simulink model "ADRC_2RD"  (Simulink 7.6)
settings: Solver=ode45  StartTime=0.0  StopTime=20  RelTol=1e-3
libraries: ADRC x3
settings Model: Creator=Administrator  LastModifiedBy=Administrator
settings DebuggingCC: AlgebraicLoopMsg=none  SolverPrmCheckMsg=none

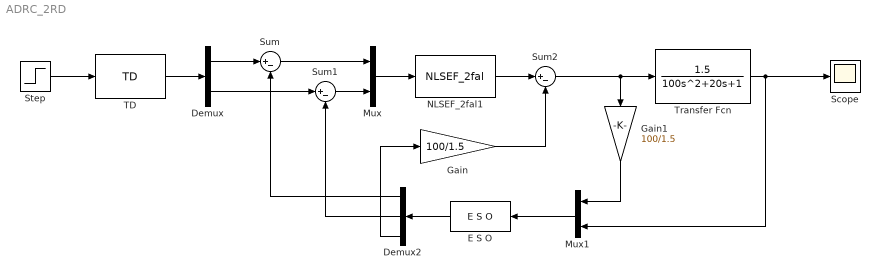
== system ADRC_2RD ==
  Demux : Demux  Outputs=2
  Demux2 : Demux  Outputs=3
  E S O : ADRC/ESO/E S O  Delta=0.1  h2=0.1  BB=[100,34,32]
  Gain : Gain  Gain=100/1.5
  Gain1 : Gain  Gain=100/1.5
  Mux : Mux  Inputs=2
  Mux1 : Mux  Inputs=2
  NLSEF_2fal1 : ADRC/NLSEF/NLSEF_2fal  Beta1=20  Beta2=30  A1=0.25  A2=0.5  Delta=0.01
  Scope : Scope
  Step : Step  Time=0  SampleTime=0
  Sum : Sum  Inputs=|+-
  Sum1 : Sum  Inputs=|+-
  Sum2 : Sum  Inputs=|+-
  TD : ADRC/TD/TD  r0=0.01  h=0.1
  Transfer Fcn : TransferFcn  Numerator=1.5  Denominator="[100 20  1]"
  wires:
  Step/1 -> TD/1
  TD/1 -> Demux/1
  Mux/1 -> NLSEF_2fal1/1
  Demux/1 -> Sum/1
  Demux/2 -> Sum1/1
  E S O/1 -> Demux2/1
  Mux1/1 -> E S O/1
  Demux2/1 -> Sum/2
  Demux2/2 -> Sum1/2
  Sum/1 -> Mux/1
  Sum1/1 -> Mux/2
  NLSEF_2fal1/1 -> Sum2/1
  Demux2/3 -> Gain/1
  Gain/1 -> Sum2/2
  Gain1/1 -> Mux1/1
  Sum2/1 -> Gain1/1, Transfer Fcn/1
  Transfer Fcn/1 -> Scope/1, Mux1/2
